simulink model "F_Simulacija_greske"  (R2016a)
settings: Solver=VariableStepAuto  StartTime=0.0  StopTime=100  RelTol=1e-3
libraries: simulink x2
settings Model: Creator=AmelT  LastModifiedBy=AmelT

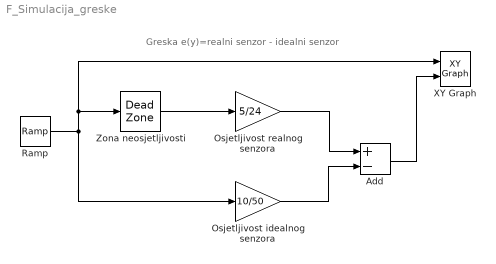
== system F_Simulacija_greske ==
  note: Greska e(y)=realni senzor - idealni senzor
  Add : Sum  Inputs=+-
  Osjetljivost idealnog senzora : Gain  Gain=10/50
  Osjetljivost realnog senzora : Gain  Gain=5/24
  Ramp : simulink/Sources/Ramp  slope=1  start=0  X0=-50
  XY Graph : simulink/Sinks/XY Graph  xmin=-50  xmax=50  ymin=-1  ymax=1  st=0.5
  Zona neosjetljivosti : DeadZone  LowerValue=-2  UpperValue=2  SaturateOnIntegerOverflow=on
  wires:
  Zona neosjetljivosti/1 -> Osjetljivost realnog senzora/1
  Add/1 -> XY Graph/2
  Ramp/1 -> Zona neosjetljivosti/1, XY Graph/1, Osjetljivost idealnog senzora/1
  Osjetljivost realnog senzora/1 -> Add/1
  Osjetljivost idealnog senzora/1 -> Add/2
